simulink model "Automatic_Control2_12"  (R2021a)
settings: Solver=VariableStepAuto  StartTime=0.0  StopTime=0.1  RelTol=1e-3
values from neighbouring files (symbols this model uses):
  b = 0.006    [Automatic_Control2.m]
  Jm = 0.05    [Automatic_Control2.m]
  Ke = 0.05    [Automatic_Control2.m]
  Kt = 0.05    [Automatic_Control2.m]
  La = 0.01    [Automatic_Control2.m]
  Ra = 10    [Automatic_Control2.m]
settings Model: Creator=Rosa  LastModifiedBy=han_jjun_mac
settings SolverCC: AlgebraicLoopSolver=TrustRegion
settings DebuggingCC: SFMachineParentedDataDiag=warning

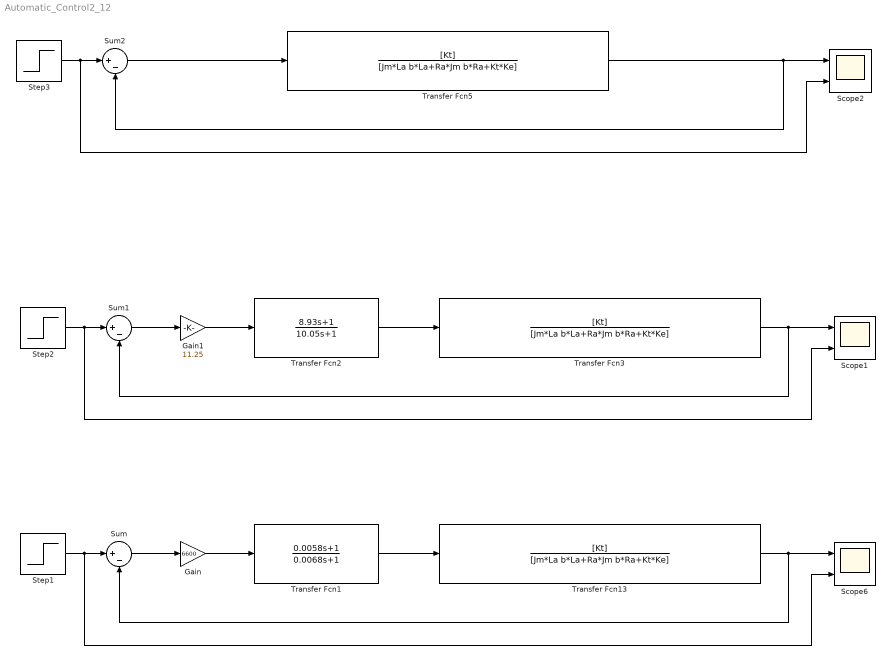
== system Automatic_Control2_12 ==
  Gain : Gain  Gain=6600
  Gain1 : Gain  Gain=11.25
  Scope1 : Scope  NumInputPorts=2
  Scope2 : Scope  NumInputPorts=2
  Scope6 : Scope  NumInputPorts=2
  Step1 : Step  Time=0  SampleTime=0
  Step2 : Step  Time=0  SampleTime=0
  Step3 : Step  Before=12  After=12  SampleTime=0
  Sum : Sum  Inputs=|+-
  Sum1 : Sum  Inputs=|+-
  Sum2 : Sum  Inputs=|+-
  Transfer Fcn1 : TransferFcn  Numerator=[0.0058 1]  Denominator=[0.0068 1]
  Transfer Fcn13 : TransferFcn  Numerator=[Kt]  Denominator=[Jm*La b*La+Ra*Jm b*Ra+Kt*Ke]
  Transfer Fcn2 : TransferFcn  Numerator=[8.93 1]  Denominator=[10.05 1]
  Transfer Fcn3 : TransferFcn  Numerator=[Kt]  Denominator=[Jm*La b*La+Ra*Jm b*Ra+Kt*Ke]
  Transfer Fcn5 : TransferFcn  Numerator=[Kt]  Denominator=[Jm*La b*La+Ra*Jm b*Ra+Kt*Ke]
  wires:
  Transfer Fcn13/1 -> Sum/2, Scope6/1
  Step1/1 -> Scope6/2, Sum/1
  Sum/1 -> Gain/1
  Gain/1 -> Transfer Fcn1/1
  Transfer Fcn1/1 -> Transfer Fcn13/1
  Transfer Fcn2/1 -> Transfer Fcn3/1
  Gain1/1 -> Transfer Fcn2/1
  Sum1/1 -> Gain1/1
  Step2/1 -> Sum1/1, Scope1/2
  Transfer Fcn3/1 -> Scope1/1, Sum1/2
  Transfer Fcn5/1 -> Scope2/1, Sum2/2
  Step3/1 -> Sum2/1, Scope2/2
  Sum2/1 -> Transfer Fcn5/1
